simulink model "ControlLoopSim"  (R2018b)
settings: Solver=FixedStepAuto  StartTime=0.0  StopTime=Tsim  FixedStep=Ts  RelTol=1e-3
values from neighbouring files (symbols this model uses):
  Ts = 0.01    [simulation.m]    (also in simulationKoop.m)
  x0 = newX    [DeltaSignal.m]    (also in simulation.m = [20/3.6; 0; 0/180*pi]; simulationKoop.m = [20/3.6; 0; 0/180*pi])
undefined symbols (not defined in the file or in its folder): nRef, nSignal, reference, steering
settings Model: Creator=Marko  LastModifiedBy=Marko

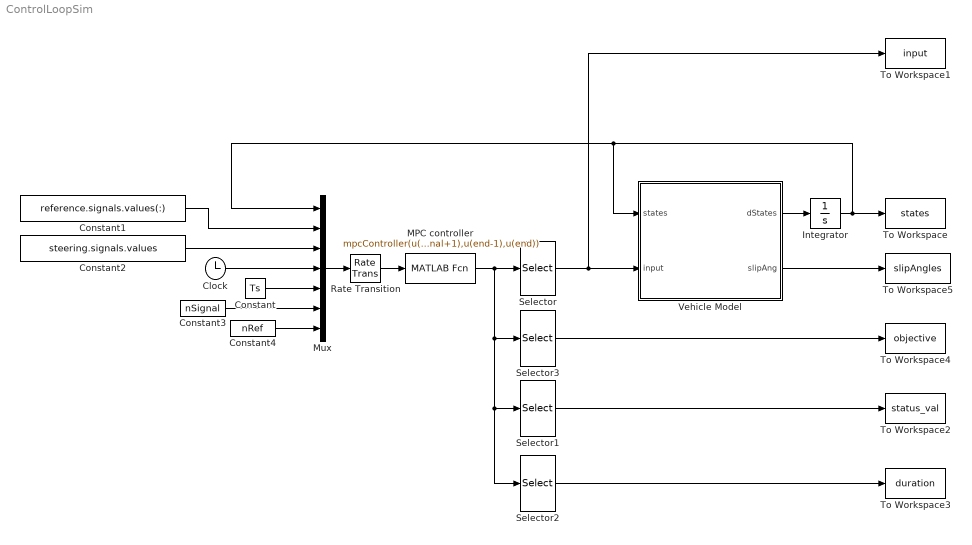
== system ControlLoopSim ==
  Clock : Clock
  Constant : Constant  Value=Ts
  Constant1 : Constant  Value=reference.signals.values(:)  SampleTime=Ts
  Constant2 : Constant  Value=steering.signals.values  SampleTime=Ts
  Constant3 : Constant  Value=nSignal
  Constant4 : Constant  Value=nRef
  Integrator : Integrator  InitialCondition=x0
  MPC controller : MATLABFcn  MATLABFcn=mpcController(u(1:3), u(4:4+nSignal*nRef-1), u(4+nSignal*nRef:4+nSignal*nRef+nSignal-1), u(4+nSignal*nRef+nSignal),u(4+nSignal*nRef+nSignal+1),u(end-1),u(end))  OutputDimensions=5 + 3
  Mux : Mux  Inputs=7
  Rate Transition : RateTransition  OutPortSampleTime=Ts
  Selector : Selector  InputPortWidth=8  IndexOptions=Index vector (dialog)  Indices=[1 2 3 4 5]  OutputSizes=1
  Selector1 : Selector  InputPortWidth=8  IndexOptions=Index vector (dialog)  Indices=7  OutputSizes=1
  Selector2 : Selector  InputPortWidth=8  IndexOptions=Index vector (dialog)  Indices=8  OutputSizes=1
  Selector3 : Selector  InputPortWidth=8  IndexOptions=Index vector (dialog)  Indices=6  OutputSizes=1
  To Workspace : ToWorkspace  VariableName=states  SaveFormat=Structure With Time  SampleTime=Ts
  To Workspace1 : ToWorkspace  VariableName=input  SaveFormat=Structure With Time  SampleTime=Ts
  To Workspace2 : ToWorkspace  VariableName=status_val  SaveFormat=Structure With Time  SampleTime=Ts
  To Workspace3 : ToWorkspace  VariableName=duration  SaveFormat=Structure With Time  SampleTime=Ts
  To Workspace4 : ToWorkspace  VariableName=objective  SaveFormat=Structure With Time  SampleTime=Ts
  To Workspace5 : ToWorkspace  VariableName=slipAngles  SaveFormat=Structure With Time  SampleTime=Ts
  Vehicle Model : MATLAB Function  TreatAsAtomicUnit=on
  wires:
  Vehicle Model/1(dStates) -> Integrator/1
  Integrator/1 -> To Workspace/1, Mux/1, Vehicle Model/1(states)
  MPC controller/1 -> Selector/1, Selector3/1, Selector2/1, Selector1/1
  Mux/1 -> Rate Transition/1
  Selector1/1 -> To Workspace2/1
  Selector/1 -> To Workspace1/1, Vehicle Model/2(input)
  Rate Transition/1 -> MPC controller/1
  Constant/1 -> Mux/5
  Clock/1 -> Mux/4
  Constant1/1 -> Mux/2
  Constant2/1 -> Mux/3
  Constant3/1 -> Mux/6
  Constant4/1 -> Mux/7
  Selector2/1 -> To Workspace3/1
  Selector3/1 -> To Workspace4/1
  Vehicle Model/2(slipAng) -> To Workspace5/1

== matlab function ControlLoopSim/Vehicle Model ==
  data: states input; dStates output; input input; slipAng output
function [dStates, slipAng] = VehicleModel(states, input)
% VEHICLE MODEL 
%   The function accepts current system states and inputs, and calculates 
%   state derivatives.

% States and input definition

vx = states(1);
vy = states(2);
omega = states(3);

deltaF = input(1);
sfl = input(2);
sfr = input(3);
srl = input(4);
srr = input(5);

% Initialize vehicle parameters
vehicle = LoadVehicleParameters();

lf = vehicle.lf;
lr = vehicle.lr;
w = vehicle.w;
m = vehicle.m;
Jz = vehicle.Jz;

% Air drag parameters
cw = vehicle.cw;
rho = vehicle.rho;
Aw = vehicle.Aw;

% VEHICLE VELOCITIES

% Longitudinal velocities
vxfl = vx - w*omega;
vxfr = vx + w*omega;
vxrl = vx - w*omega;
vxrr = vx + w*omega;
% Lateral velocities
vyfl = vy + lf*omega;
vyfr = vy + lf*omega;
vyrl = vy - lr*omega;
vyrr = vy - lr*omega;

% TYRE VELOCITIES

% Longitudinal velocities
vlfl = vxfl*cos(deltaF) + vyfl*sin(deltaF);
vlfr = vxfr*cos(deltaF) + vyfr*sin(deltaF);
vlrl = vxrl;
vlrr = vxrr;

% Cornering velocities
vcfl = -vxfl*sin(deltaF) + vyfl*cos(deltaF);
vcfr = -vxfr*sin(deltaF) + vyfr*cos(deltaF);
vcrl = vyrl;
vcrr = vyrr;

% TYRE SLIP ANGLES
alpha_fl = atan2(vcfl,vlfl);
alpha_fr = atan2(vcfr,vlfr);
alpha_rl = atan2(vcrl,vlrl);
alpha_rr = atan2(vcrr,vlrr);

% TYRE FORCES
Cx = vehicle.Cx;
Cy = vehicle.Cy;

% Longitudinal forces
Flfl = Cx*sfl;
Flfr = Cx*sfr;
Flrl = Cx*srl;
Flrr = Cx*srr;

% Conrnering forces
Fcfl = -Cy*alpha_fl;
Fcfr = -Cy*alpha_fr;
Fcrl = -Cy*alpha_rl;
Fcrr = -Cy*alpha_rr;

% AXLE FORCES

% Longitudinal forces
Fxfl = Flfl*cos(deltaF) - Fcfl*sin(deltaF);
Fxfr = Flfr*cos(deltaF) - Fcfr*sin(deltaF);
Fxrl = Flrl;
Fxrr = Flrr;

% Lateral forces
Fyfl = Flfl*sin(deltaF) + Fcfl*cos(deltaF);
Fyfr = Flfr*sin(deltaF) + Fcfr*cos(deltaF);
Fyrl = Fcrl;
Fyrr = Fcrr;

% VEHICLE DYNAMICS MODEL

dvx = vy*omega + 1/m*(-0.5*cw*rho*Aw*sqrt(vx^2+vy^2)*vx + Fxfl + Fxfr + Fxrl + Fxrr);
dvy = -vx*omega + 1/m*(-0.5*cw*rho*Aw*sqrt(vx^2+vy^2)*vy + Fyfl + Fyfr + Fyrl + Fyrr);
dOmega = lf/Jz*(Fyfl + Fyfr) - lr/Jz*(Fyrl + Fyrr) + w/Jz*(-Fxfl + Fxfr -Fxrl + Fxrr);

dStates = [dvx; dvy; dOmega];
slipAng = [alpha_fl; alpha_fr; alpha_rl; alpha_rr];
end
